simulink model "FMS"  (R2018b)
settings: configuration reference "FMS_config" (kept outside this file)
values from neighbouring files (symbols this model uses):
  FMS_EXPORT = Simulink.Parameter(FMS_EXPORT_VALUE)    [base_fms_var.m]
  FMS_PARAM = Simulink.Parameter(FMS_PARAM_VALUE)    [base_fms_var.m]
undefined symbols (not defined in the file or in its folder): actuator_cmd, DiscIntNeverNeededParam, mode, p_cmd, phi_cmd, psi_rate_cmd, q_cmd, r_cmd, reset, state, theta_cmd, throttle_cmd, timestamp, u_cmd, v_cmd, w_cmd
libraries: simulink x39, Rotation x2, Filter x1
(part 2 of 2)

== system FMS/Control_Mode/Altitude_Hold_Mode/Command_Generator/Vel_Command/Subsystem1/Height_Control/Position_Error ==
  INS_Out : Inport
  motion_state : Inport  Port=2
  Bus_Selection : Subsystem
  Compare To Constant1 : simulink/Logic and Bit Operations/Compare To Constant  relop===  const=2  OutDataTypeStr=boolean
  Detect Increase1 : simulink/Logic and Bit Operations/Detect Increase  vinit=0.0  OutDataTypeStr=boolean
  Sum : Sum  Inputs=-+|
  Z_Holder : Subsystem
  pos_z_err_R_C : Outport
  wires:
  Z_Holder/1(y) -> Sum/2  "hold_z"
  Detect Increase1/1 -> Z_Holder/2(update)
  Compare To Constant1/1 -> Detect Increase1/1
  motion_state/1 -> Compare To Constant1/1
  Sum/1 -> pos_z_err_R_C/1
  INS_Out/1 -> Bus_Selection/1(INS_Out)
  Bus_Selection/1(pos_z_O) -> Sum/1, Z_Holder/1(u)  "pos_z"

== system FMS/Control_Mode/Manual_Mode/Command_Generator/Psi_Rate_Command/Heading_Control/Heading_Error/Bus_Selection ==
  INS_Out : Inport
  Bus Selector2 : BusSelector  OutputSignals=psi
  psi_rad : Outport
  wires:
  Bus Selector2/1 -> psi_rad/1  "<psi>"
  INS_Out/1 -> Bus Selector2/1

== system FMS/Control_Mode/Manual_Mode/Command_Generator/Psi_Rate_Command/Heading_Control/Heading_Error/Holder ==
  u : Inport
  update : Inport  Port=2
  Delay : Delay  DelayLength=1  InitialConditionSource=Input port
      settings: InputPortMap=u0,p4
  Switch1 : Switch  Criteria=u2 > Threshold
  y : Outport
  wires:
  u/1 -> Delay/2, Switch1/1
  update/1 -> Switch1/2
  Delay/1 -> Switch1/3
  Switch1/1 -> Delay/1, y/1

== system FMS/Control_Mode/Position_Mode/Command_Generator/Psi_Rate_Command/Heading_Control/Heading_Error/Bus_Selection ==
  INS_Out : Inport
  Bus Selector2 : BusSelector  OutputSignals=psi
  psi_rad : Outport
  wires:
  INS_Out/1 -> Bus Selector2/1
  Bus Selector2/1 -> psi_rad/1  "<psi>"

== system FMS/Control_Mode/Position_Mode/Command_Generator/Psi_Rate_Command/Heading_Control/Heading_Error/Holder ==
  u : Inport
  update : Inport  Port=2
  Delay : Delay  DelayLength=1  InitialConditionSource=Input port
      settings: InputPortMap=u0,p4
  Switch1 : Switch  Criteria=u2 > Threshold
  y : Outport
  wires:
  Switch1/1 -> y/1, Delay/1
  Delay/1 -> Switch1/3
  update/1 -> Switch1/2
  u/1 -> Delay/2, Switch1/1

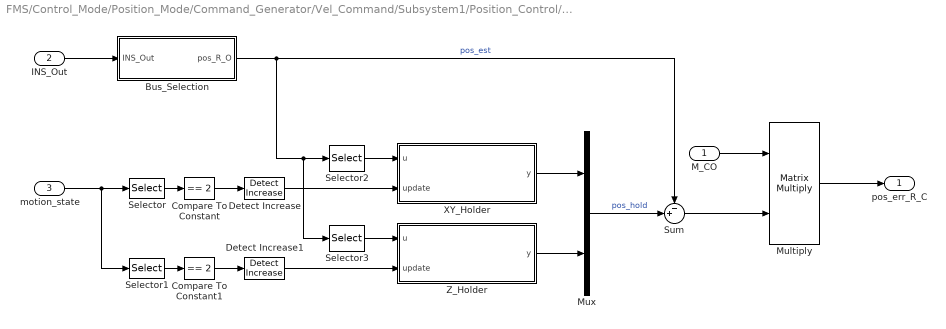
== system FMS/Control_Mode/Position_Mode/Command_Generator/Vel_Command/Subsystem1/Position_Control/Position_Error ==
  M_CO : Inport
  INS_Out : Inport  Port=2
  motion_state : Inport  Port=3
  Bus_Selection : Subsystem
  Compare To Constant : simulink/Logic and Bit Operations/Compare To Constant  relop===  const=2  OutDataTypeStr=boolean
  Compare To Constant1 : simulink/Logic and Bit Operations/Compare To Constant  relop===  const=2  OutDataTypeStr=boolean
  Detect Increase : simulink/Logic and Bit Operations/Detect Increase  vinit=0.0  OutDataTypeStr=boolean
  Detect Increase1 : simulink/Logic and Bit Operations/Detect Increase  vinit=0.0  OutDataTypeStr=boolean
  Multiply : Product  Multiplication=Matrix(*)
  Mux : Mux  Inputs=2
  Selector : Selector  InputPortWidth=2  IndexOptions=Index vector (dialog)  Indices=1  OutputSizes=1
  Selector1 : Selector  InputPortWidth=2  IndexOptions=Index vector (dialog)  Indices=2  OutputSizes=1
  Selector2 : Selector  InputPortWidth=3  IndexOptions=Index vector (dialog)  Indices=[1 2]  OutputSizes=1
  Selector3 : Selector  InputPortWidth=3  IndexOptions=Index vector (dialog)  Indices=3  OutputSizes=1
  Sum : Sum  Inputs=-+|
  XY_Holder : Subsystem
  Z_Holder : Subsystem
  pos_err_R_C : Outport
  wires:
  Mux/1 -> Sum/2  "pos_hold"
  Z_Holder/1(y) -> Mux/2
  Selector3/1 -> Z_Holder/1(u)
  Selector2/1 -> XY_Holder/1(u)
  Detect Increase1/1 -> Z_Holder/2(update)
  Compare To Constant1/1 -> Detect Increase1/1
  Detect Increase/1 -> XY_Holder/2(update)
  Selector1/1 -> Compare To Constant1/1
  Compare To Constant/1 -> Detect Increase/1
  Selector/1 -> Compare To Constant/1
  M_CO/1 -> Multiply/1
  Multiply/1 -> pos_err_R_C/1
  XY_Holder/1(y) -> Mux/1
  INS_Out/1 -> Bus_Selection/1(INS_Out)
  motion_state/1 -> Selector/1, Selector1/1
  Sum/1 -> Multiply/2
  Bus_Selection/1(pos_R_O) -> Selector2/1, Selector3/1, Sum/1  "pos_est"

== system FMS/Control_Mode/Altitude_Hold_Mode/Command_Generator/Vel_Command/Subsystem1/Height_Control/Position_Error/Bus_Selection ==
  INS_Out : Inport
  Bus Selector2 : BusSelector  OutputSignals=h_R
  Gain : Gain  Gain=-1
  pos_z_O : Outport
  wires:
  Gain/1 -> pos_z_O/1
  Bus Selector2/1 -> Gain/1  "<h_R>"
  INS_Out/1 -> Bus Selector2/1

== system FMS/Control_Mode/Altitude_Hold_Mode/Command_Generator/Vel_Command/Subsystem1/Height_Control/Position_Error/Z_Holder ==
  u : Inport
  update : Inport  Port=2
  Delay : Delay  DelayLength=1  InitialConditionSource=Input port
      settings: InputPortMap=u0,p4
  Switch1 : Switch  Criteria=u2 > Threshold
  y : Outport
  wires:
  Switch1/1 -> y/1, Delay/1
  Delay/1 -> Switch1/3
  update/1 -> Switch1/2
  u/1 -> Delay/2, Switch1/1

== system FMS/Control_Mode/Position_Mode/Command_Generator/Vel_Command/Subsystem1/Position_Control/Position_Error/Bus_Selection ==
  INS_Out : Inport
  Bus Selector2 : BusSelector  OutputSignals=x_R,y_R,h_R
  Gain : Gain  Gain=-1
  Mux3 : Mux  Inputs=3
  pos_R_O : Outport
  wires:
  Mux3/1 -> pos_R_O/1
  Gain/1 -> Mux3/3
  Bus Selector2/1 -> Mux3/1  "<x_R>"
  Bus Selector2/2 -> Mux3/2  "<y_R>"
  Bus Selector2/3 -> Gain/1  "<h_R>"
  INS_Out/1 -> Bus Selector2/1

== system FMS/Control_Mode/Position_Mode/Command_Generator/Vel_Command/Subsystem1/Position_Control/Position_Error/XY_Holder ==
  u : Inport
  update : Inport  Port=2
  Delay : Delay  DelayLength=1  InitialConditionSource=Input port
      settings: InputPortMap=u0,p4
  Switch1 : Switch  Criteria=u2 > Threshold
  y : Outport
  wires:
  u/1 -> Delay/2, Switch1/1
  update/1 -> Switch1/2
  Delay/1 -> Switch1/3
  Switch1/1 -> Delay/1, y/1

== system FMS/Control_Mode/Position_Mode/Command_Generator/Vel_Command/Subsystem1/Position_Control/Position_Error/Z_Holder ==
  u : Inport
  update : Inport  Port=2
  Delay : Delay  DelayLength=1  InitialConditionSource=Input port
      settings: InputPortMap=u0,p4
  Switch1 : Switch  Criteria=u2 > Threshold
  y : Outport
  wires:
  Switch1/1 -> y/1, Delay/1
  Delay/1 -> Switch1/3
  update/1 -> Switch1/2
  u/1 -> Delay/2, Switch1/1

== stateflow chart FMS/Control_Mode/Mode_Logic ==
  state Unknow
    entry:
    local_mode = 0;
  state Mission
    entry:
    local_mode = 1;
  state Position
    entry:
    local_mode = 2;
  state Altitude_Hold
    entry:
    local_mode = 3;
  state Manual
    entry:
    local_mode = 4;
  state Acro
    entry:
    local_mode = 5;
  (junction 126) -> Unknow
  Unknow -> (junction 130)
  (junction 115) -> (junction 126) [order 2]
  (junction 130) -> (junction 75)
  (junction 115) -> Mission [order 1] : [mode == 1]
  Mission -> (junction 73)
  (junction 73) -> (junction 75) [order 1] : [bitget(flag, 4) && bitget(flag, 6)]
  (junction 50) -> (junction 115) [order 2]
  (junction 73) -> Position [order 2]
  (junction 75) -> (junction 81)
  (junction 50) -> Position [order 1] : [mode == 2]
  Position -> (junction 79)
  (junction 79) -> (junction 81) [order 1] : [bitget(flag, 4) && bitget(flag, 7) && bitget(flag, 8)]
  (junction 53) -> (junction 50) [order 2]
  (junction 79) -> Altitude_Hold [order 2]
  (junction 81) -> (junction 90)
  (junction 53) -> Altitude_Hold [order 1] : [mode == 3]
  Altitude_Hold -> (junction 88)
  (junction 88) -> (junction 90) [order 1] : [bitget(flag, 8)]
  (junction 56) -> (junction 53) [order 2]
  (junction 88) -> Manual [order 2]
  (junction 90) -> (junction 98)
  (junction 56) -> Manual [order 1] : [mode == 4]
  Manual -> (junction 136)
  (junction 136) -> (junction 98) [order 1] : [bitget(flag, 3)]
  (junction 59) -> (junction 56) [order 2]
  (junction 136) -> Acro [order 2]
  (junction 98) -> (junction 103)
  (default) -> (junction 59)
  (junction 59) -> Acro [order 1] : [mode == 5]
  Acro -> (junction 103)
  (junction 108) -> (junction 59)
  (junction 103) -> (junction 106)
  (junction 106) -> (junction 108) : {control_mode = local_mode;}
  data: mode input; local_mode local uint32; flag input uint32; control_mode output

== stateflow chart FMS/Control_Mode/Altitude_Hold_Mode/Command_Generator/Psi_Rate_Command/Motion_State ==
  state Hold
    entry:
    state=2;
  state Move
    entry:
    state=0;
  state Brake
    entry:
    state=1;
  (default) -> Move
  Hold -> Move : [move_cmd==1]
  Move -> Brake : [move_cmd==0]
  Brake -> Move [order 2] : [move_cmd==1]
  Brake -> Hold [order 1] : [heading_rate<=0.1 || after(1, sec)]
  data: move_cmd input; heading_rate input; state output

== stateflow chart FMS/State_Management/Arm_Event/Arm_Event ==
  state Idle
    en:
    arm_event = 0;
  state arm_event
    en:
    arm_event = 1;
  state ready
  (default) -> Idle
  arm_event -> Idle
  Idle -> ready : [stick_throttle < -0.8 && stick_roll < -0.8 && stick_pitch < -0.8]
  ready -> arm_event : [abs(stick_roll) < 0.15 && abs(stick_pitch)<0.15]
  data: stick_roll input; stick_pitch input; stick_throttle input; arm_event output

== stateflow chart FMS/State_Management/State_Logic ==
  state Motor_Test
    entry:
    State = 1;
    during:
    PWM_Cmd = 1000 + uint16((Stick_Throttle+1)*500);
  state Disarm
    entry:
    State = 0;
    PWM_Cmd = 1000;
  state Arm
    entry:
    State = 2;
  state Standby
    entry:
    State = 1;
    PWM_Cmd = 1100;
  Disarm -> Motor_Test [order 1] : [Test_Motor == 1 && Arm_Event == 1]
  Motor_Test -> Disarm : [Test_Motor == 0 || Arm_Event == 1]
  (default) -> Disarm
  Arm -> Disarm [order 1] : [Disarm_Event == 1 && Disarm_Allowed == 1]
  Arm -> Disarm [order 2] : [Force_Disarm]
  Disarm -> Standby [order 2] : [Arm_Event == 1 && Arm_Allowed == 1]
  Standby -> Disarm [order 1] : after(30,sec)
  Standby -> Disarm [order 3] : [Arm_Event == 1 || Force_Disarm]
  Standby -> Arm [order 2] : [Stick_Throttle > -0.25]
  data: PWM_Cmd output uint16; State output; Arm_Allowed input; Disarm_Allowed input; Arm_Event input; Disarm_Event input; Stick_Throttle input; Force_Disarm input; Test_Motor input

== stateflow chart FMS/Control_Mode/Position_Mode/Command_Generator/Psi_Rate_Command/Motion_State ==
  state Hold
    entry:
    state=2;
  state Move
    entry:
    state=0;
  state Brake
    entry:
    state=1;
  (default) -> Move
  Hold -> Move : [move_cmd==1]
  Move -> Brake : [move_cmd==0]
  Brake -> Move [order 2] : [move_cmd==1]
  Brake -> Hold [order 1] : [heading_rate<=0.1 || after(1, sec)]
  data: move_cmd input; heading_rate input; state output

== stateflow chart FMS/Control_Mode/Manual_Mode/Command_Generator/Psi_Rate_Command/Motion_State ==
  state Hold
    entry:
    state=2;
  state Move
    entry:
    state=0;
  state Brake
    entry:
    state=1;
  (default) -> Move
  Hold -> Move : [move_cmd==1]
  Move -> Brake : [move_cmd==0]
  Brake -> Move [order 2] : [move_cmd==1]
  Brake -> Hold [order 1] : [heading_rate<=0.1 || after(1, sec)]
  data: move_cmd input; heading_rate input; state output

== stateflow chart FMS/Control_Mode/Position_Mode/Command_Generator/Vel_Command/Motion_State/XY_Motion_State ==
  state Hold
    entry:
    state=2;
  state Move
    entry:
    state=0;
  state Brake
    entry:
    state=1;
  (default) -> Move
  Hold -> Move : [move_cmd==1]
  Move -> Brake : [move_cmd==0]
  Brake -> Move [order 2] : [move_cmd==1]
  Brake -> Hold [order 1] : [speed<=0.2 || after(2.5, sec)]
  data: move_cmd input; state output; speed input

== stateflow chart FMS/Control_Mode/Position_Mode/Command_Generator/Vel_Command/Motion_State/Z_Motion_State ==
  state Hold
    entry:
    state=2;
  state Move
    entry:
    state=0;
  state Brake
    entry:
    state=1;
  (default) -> Move
  Hold -> Move : [move_cmd==1]
  Move -> Brake : [move_cmd==0]
  Brake -> Move [order 2] : [move_cmd==1]
  Brake -> Hold [order 1] : [abs(speed)<=0.2 || after(1.5, sec)]
  data: move_cmd input; state output; speed input

== stateflow chart FMS/Control_Mode/Altitude_Hold_Mode/Command_Generator/Vel_Command/Motion_State/Z_Motion_State ==
  state Hold
    entry:
    state=2;
  state Move
    entry:
    state=0;
  state Brake
    entry:
    state=1;
  (default) -> Move
  Hold -> Move : [move_cmd==1]
  Move -> Brake : [move_cmd==0]
  Brake -> Move [order 2] : [move_cmd==1]
  Brake -> Hold [order 1] : [abs(speed)<=0.2 || after(1.5, sec)]
  data: move_cmd input; state output; speed input

== stateflow chart FMS/State_Management/Arm_Event/Disarm_Event ==
  state Disarm
    en:
    disarm_event = 1;
  state Idle
    en:
    disarm_event = 0;
  state On_Ground
  (default) -> Idle
  Disarm -> Idle
  On_Ground -> Disarm [order 2] : [after(1.5, sec)]
  On_Ground -> Idle [order 1] : [on_ground == 0]
  Idle -> On_Ground : [on_ground == 1 && state == 2]
  data: on_ground input; disarm_event output; state input
